simulink model "lidarMapping"  (R2022b)
settings: Solver=FixedStepAuto  StartTime=0.0  StopTime=100  FixedStep=0.01  RelTol=1e-3
InitFcn:
  | Ts = 0.01;
libraries: instrumentseriallib x2, visionsinks x1
settings Model: Creator=System-10  LastModifiedBy=System-10
settings ModelReferenceCC: PropagateVarSize=Only when enabling

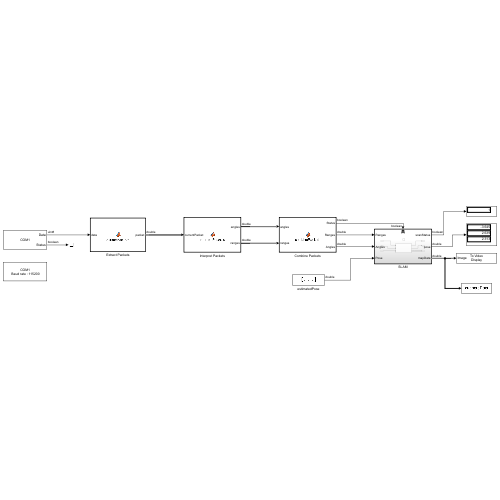
[thumbnail: Simulink's stored preview of the top-level diagram]
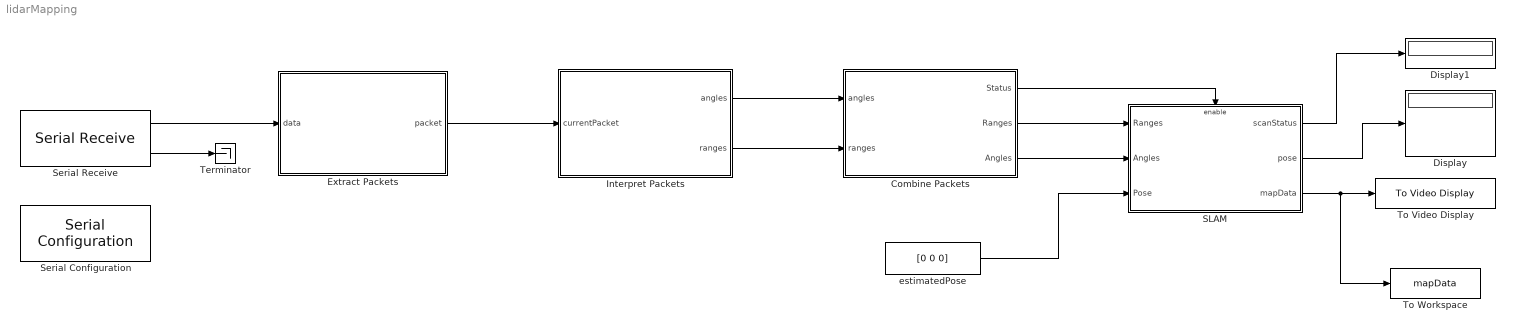
== system lidarMapping ==
  Combine Packets : MATLAB Function  TreatAsAtomicUnit=on
  Display : Display
  Display1 : Display
  Extract Packets : MATLAB Function  TreatAsAtomicUnit=on
  Interpret Packets : MATLAB Function  TreatAsAtomicUnit=on
  SLAM : Subsystem
  Serial Configuration : instrumentseriallib/Serial Configuration  Priority=-200000  PortSel=COM1  Port=COM1  ComPort=COM1  BaudRate=115200  DataBits=8  Parity=none  StopBits=1  ByteOrder=little-endian  FlowControl=none  Timeout=10  SimulateUsing=Interpreted execution  BlockInModel=on  aMode=1
  Serial Receive : instrumentseriallib/Serial Receive  Priority=1  PortSel=COM1  Port=COM1  ComPort=COM1  DataType=uint8  SaveDataType=uint8  ToggleHeader=off  Header=[170 85]  ToggleTerminator=off  Terminator=<none>  CustomTerminator=[]  InputFormat=Column major  ToggleDataSize=on  DataSize=[1 2000]  EnableBlockingMode=off  ActionDataUnavailable=Output last received value  ActionWhenDataUnavailable=Output last received value  CustomValue=111  SampleTime=Ts  SimulateUsing=Interpreted execution  BlockInModel=on  aMode=1
  Terminator : Terminator
  To Video Display : visionsinks/To Video Display  windowSizeMode=Normal  openAtMdlStart=on  fullScreen=off  videoWindowX=536805376  videoWindowY=536805376  saveWindowSize=off  videoWindowWidth=1000  videoWindowHeight=1000  inputColorFormat=RGB  inputType=Obsolete  imagePorts=One multidimensional signal  OutputDevice=On-screen video monitor  dataOrg=Column-major  isWindowOpen=off
  To Workspace : ToWorkspace  VariableName=mapData  SaveFormat=Timeseries  SampleTime=Ts
  estimatedPose : Constant  Value=[0 0 0]
  wires:
  Serial Receive/1 -> Extract Packets/1(data)
  Extract Packets/1(packet) -> Interpret Packets/1(currentPacket)
  Serial Receive/2 -> Terminator/1
  Interpret Packets/1(angles) -> Combine Packets/1(angles)
  Interpret Packets/2(ranges) -> Combine Packets/2(ranges)
  Combine Packets/2(Ranges) -> SLAM/1(Ranges)
  Combine Packets/3(Angles) -> SLAM/2(Angles)
  Combine Packets/1(Status) -> SLAM/Enable
  SLAM/3(mapData) -> To Video Display/1, To Workspace/1
  estimatedPose/1 -> SLAM/3(Pose)
  SLAM/2(pose) -> Display/1
  SLAM/1(scanStatus) -> Display1/1

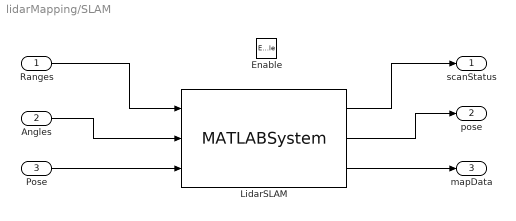
== system lidarMapping/SLAM ==
  Ranges : Inport
  Angles : Inport  Port=2
  Pose : Inport  Port=3
  Enable : EnablePort  PropagateVarSize=During execution
  LidarSLAM : MATLABSystem  System=LidarSlam_interp  SimulateUsing=Interpreted execution
      mask Type: LidarSlam_interp
      mask Display:
      | disp('LidarSlam_interp');
      | port_label('input',1,'ranges');
      | port_label('input',2,'angles');
      | port_label('input',3,'relPoseEst');
      | port_label('output',1,'isScanAdded');
      | port_label('output',2,'pose');
      | port_label('output',3,'mapData');
  scanStatus : Outport
  pose : Outport  Port=2
  mapData : Outport  Port=3
  wires:
  Ranges/1 -> LidarSLAM/1
  Angles/1 -> LidarSLAM/2
  LidarSLAM/2 -> pose/1
  LidarSLAM/1 -> scanStatus/1
  LidarSLAM/3 -> mapData/1
  Pose/1 -> LidarSLAM/3

== matlab function lidarMapping/Extract Packets ==
  settings: updateMethod=DISCRETE  sampleTime=Ts
  data: data input; packet output double size=[1 90]
function packet = extractPackets(data)
    persistent indicesOfHeaders;
    persistent startIdx;
    persistent endIdx;
    persistent idx;
    persistent lastData;

    if isempty(lastData)
        lastData = uint8(zeros(1,size(data,2)));
    end

    if isempty(indicesOfHeaders) || ~isequal(data, lastData)
        
        indicesOfAA = find(data == 170);
        indicesOfHeaders = zeros(1, length(indicesOfAA)); 
        count = 0;
        
        startIdx = 0;
        endIdx = 0;
        idx = 0;

        for i = 1:length(indicesOfAA)
            if indicesOfAA(i) < length(data) && data(indicesOfAA(i) + 1) == 85
                count = count + 1;
                indicesOfHeaders(count) = indicesOfAA(i);
            end
        end

        indicesOfHeaders = indicesOfHeaders(1:count);
        lastData = data;      
    end
    
    if ~(isempty(indicesOfHeaders))
        if endIdx < indicesOfHeaders(end)
            idx = idx + 1;
            startIdx = indicesOfHeaders(idx);
            endIdx = indicesOfHeaders(idx+1);
            packet = double(data(startIdx:endIdx-1));
        else
            packet = [];
        end
    else
        packet = [];
    end
end

== matlab function lidarMapping/Interpret Packets ==
  settings: updateMethod=DISCRETE  sampleTime=Ts
  data: currentPacket input; angles output size=[1 40]; ranges output size=[1 40]
function [angles, ranges] = interpretPackets(currentPacket)

    if size(currentPacket, 2) < 90
        angles = [];
        ranges = [];
        return;
    end

    FSA = double(bitor(bitshift(uint16(currentPacket(1, 6)), 8), uint16(currentPacket(1, 5)), 'uint16'));
    LSA = double(bitor(bitshift(uint16(currentPacket(1, 8)), 8), uint16(currentPacket(1, 7)), 'uint16'));
    
    AngleFSA = double(bitshift(FSA, -1) / 64);
    AngleLSA = double(bitshift(LSA, -1) / 64);
    diffAngle = mod((AngleLSA - AngleFSA),360);
    
    rawSi = uint8(currentPacket(:, 11:end));
    
    Si = zeros(1, 40);
    for i = 1:2:length(rawSi)
        Si((i + 1) / 2) = double(bitor(bitshift(uint16(rawSi(1, i + 1)), 8), uint16(rawSi(1, i)), 'uint16'));
    end
    
    AngleSi = zeros(1, 40);
    if Si(1) == 0
        AngleSi(1) = AngleFSA;
    else
        AngleSi(1) = AngleFSA + atan(21.8*((155.3-Si(1))/(155.3*Si(1))));
    end

    for i = 2:39
        if Si(i) == 0
            AngleSi(i) = ((diffAngle / (40 - 1)) * (i - 1) + AngleFSA);
        else
            AngleSi(i) = ((diffAngle / (40 - 1)) * (i - 1) + AngleFSA) + atan(21.8*((155.3-Si(i))/(155.3*Si(i))));
        end
    end

    if Si(40) == 0
        AngleSi(40) = AngleLSA;
    else
        AngleSi(40) = AngleLSA + atan(21.8*((155.3-Si(end))/(155.3*Si(end))));
    end

    %Current Angles as 1x40 array [deg].
    angles = AngleSi;

    %Current Ranges as 1x40 array [meter].
    Si = Si / 4000;
    ranges = Si;
end

== matlab function lidarMapping/Combine Packets ==
  settings: updateMethod=DISCRETE  sampleTime=Ts
  data: Status output boolean; Ranges output size=[1 400]; angles input; Angles output size=[1 400]; ranges input
function [Status,Ranges,Angles]  = combinePackets(angles,ranges)
    persistent count; 
    persistent elemAngles;
    persistent elemRanges;

    if isempty(count)
        count = 0;
        elemAngles = zeros(1,400);
        elemRanges = zeros(1,400);
    end
        
    for i = 1:length(angles)
        elemAngles(i+count) = angles(i);
        elemRanges(i+count) = ranges(i);
    end
    if count < (length(elemAngles)-length(angles))
        count = count + length(angles);
        Angles = zeros(1,400);
        Ranges = zeros(1,400);
        Status = boolean(0);
    else
        count = 0;
        %Current Angles as 1x400 array [rad].
        Angles = deg2rad(elemAngles);
        %Current Ranges as 1x400 array [meter].
        Ranges = elemRanges;
        Status = boolean(1);
    end
end
